simulink model "a01_SimTurret"  (R2024a)
settings: Solver=VariableStepAuto  StartTime=0.0  StopTime=10  FixedStep=0.000001  MaxStep=mSim.dTime*0.01  RelTol=mSim.dTime*0.01
PostLoadFcn:
  | a02_SimVariable
undefined symbols (not defined in the file): A02MTRPA, a1st, B01SCHED, b5th, C01ISENS, c7th, CRX1, DC, E03LIM, H01MDE, H01TRT, Init, mDefine, Mech, mSim, MtrPar, Sim, SIM, SimMde
libraries: spsSeriesRLCBranchLib x17, simulink x8, spsCurrentMeasurementLib x7, spsIGBTDiodeLib x7, spsDiodeLib x6, spsControlledVoltageSourceLib x6, spsVoltageMeasurementLib x4, SignalEditorBlockLib x3, spsDCVoltageSourceLib x1, spspowerguiLib x1
(part 2 of 3)

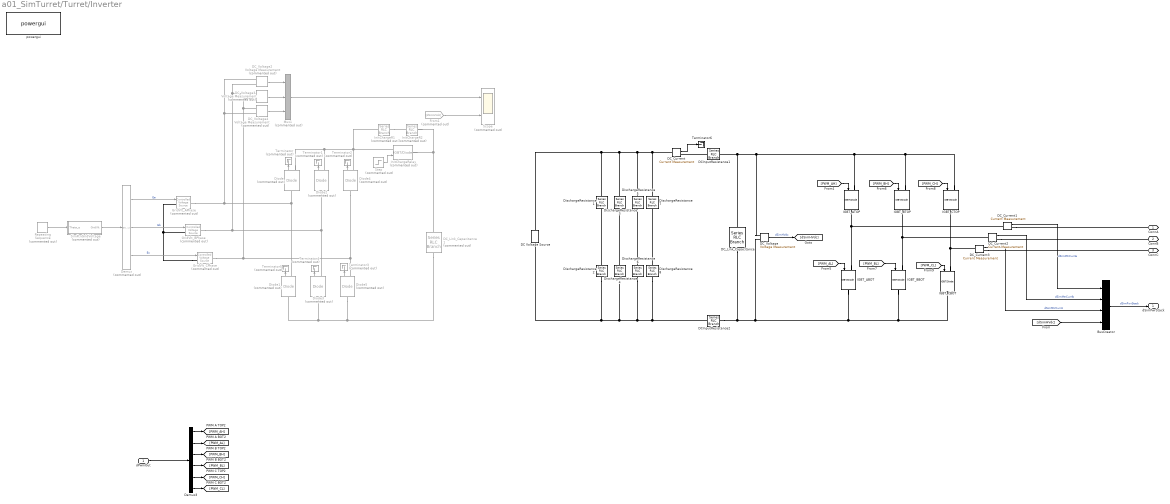
== system a01_SimTurret/Turret/Inverter ==
  dPwmOut : Inport
  BusCreator : BusCreator  Inputs=4
  DC Voltage Source : spsDCVoltageSourceLib/DC Voltage Source  Amplitude=Sim.dInitHVdc  Measurements=None
  DCInputResistance1 : spsSeriesRLCBranchLib/Series RLC Branch  LConnTagsString=__new0  RConnTagsString=__new0  BranchType=R  Resistance=1e-3  Inductance=1e-6  SetiL0=off  InitialCurrent=0  Capacitance=1e-6  Setx0=off  InitialVoltage=0  Measurements=None
  DCInputResistance2 : spsSeriesRLCBranchLib/Series RLC Branch  LConnTagsString=__new0  RConnTagsString=__new0  BranchType=R  Resistance=1e-3  Inductance=1e-6  SetiL0=off  InitialCurrent=0  Capacitance=1e-6  Setx0=off  InitialVoltage=0  Measurements=None
  DC_Current{,1..3} (4 alike) : spsCurrentMeasurementLib/Current Measurement  PhasorSimulation=off  OutputType=Complex  PSBequivalent=0
  DC_Link_Capacitance : spsSeriesRLCBranchLib/Series RLC Branch  LConnTagsString=__new0  RConnTagsString=__new0  BranchType=C  Resistance=DC.Rout  Inductance=1e-3  SetiL0=off  InitialCurrent=0  Capacitance=Sim.Dc.Capacitance  Setx0=on  InitialVoltage=Sim.dInitHVdc  Measurements=None
  DC_Link_Capacitance1 : spsSeriesRLCBranchLib/Series RLC Branch  Commented=on  LConnTagsString=__new0  RConnTagsString=__new0  BranchType=C  Resistance=DC.Rout  Inductance=1e-3  SetiL0=off  InitialCurrent=0  Capacitance=Sim.Dc.Capacitance  Setx0=on  InitialVoltage=Sim.dInitHVdc  Measurements=None
  DC_Voltage : spsVoltageMeasurementLib/Voltage Measurement  PhasorSimulation=off  OutputType=Complex  PSBequivalent=0
  DC_Voltage2 : spsVoltageMeasurementLib/Voltage Measurement  Commented=on  PhasorSimulation=off  OutputType=Complex  PSBequivalent=0
  DC_Voltage3 : spsVoltageMeasurementLib/Voltage Measurement  Commented=on  PhasorSimulation=off  OutputType=Complex  PSBequivalent=0
  DC_Voltage4 : spsVoltageMeasurementLib/Voltage Measurement  Commented=on  PhasorSimulation=off  OutputType=Complex  PSBequivalent=0
  Demux : Demux  Commented=on  Outputs=3
  Demux3 : Demux  Outputs=6
  Diode{,1..5} (6 alike) : spsDiodeLib/Diode  Commented=on  Ron=0.001  Lon=0  Vf=0.8  IC=0  UseSnubber=0  Rs=500  Cs=250e-9  Measurements=on
  DischargeResistance{1..8} (8 alike) : spsSeriesRLCBranchLib/Series RLC Branch  LConnTagsString=__new0  RConnTagsString=__new0  BranchType=R  Resistance=Sim.Dc.DischargeR  Inductance=1e-3  SetiL0=off  InitialCurrent=0  Capacitance=1e-6  Setx0=off  InitialVoltage=0  Measurements=None
  From1 : From  Commented=on  GotoTag=dSimHVdc
  GridVlt_APhase : spsControlledVoltageSourceLib/Controlled Voltage Source  Commented=on  Initialize=off  Source_Type=DC  Amplitude=0  Phase=0  Frequency=0  Measurements=None
  GridVlt_BPhase : spsControlledVoltageSourceLib/Controlled Voltage Source  Commented=on  Initialize=off  Source_Type=DC  Amplitude=0  Phase=0  Frequency=0  Measurements=None
  GridVlt_CPhase : spsControlledVoltageSourceLib/Controlled Voltage Source  Commented=on  Initialize=off  Source_Type=DC  Amplitude=0  Phase=0  Frequency=0  Measurements=None
  IGBT_ABOT : spsIGBTDiodeLib/IGBT//Diode  Ron=Sim.Igbt.Ron  Rs=Sim.Igbt.Roff  Cs=Sim.Igbt.Csnb  Measurements=off
  IGBT_ATOP : spsIGBTDiodeLib/IGBT//Diode  Ron=Sim.Igbt.Ron  Rs=Sim.Igbt.Roff  Cs=Sim.Igbt.Csnb  Measurements=off
  IGBT_BBOT : spsIGBTDiodeLib/IGBT//Diode  Ron=Sim.Igbt.Ron  Rs=Sim.Igbt.Roff  Cs=Sim.Igbt.Csnb  Measurements=off
  IGBT_BTOP : spsIGBTDiodeLib/IGBT//Diode  Ron=Sim.Igbt.Ron  Rs=Sim.Igbt.Roff  Cs=Sim.Igbt.Csnb  Measurements=off
  IGBT_CBOT : spsIGBTDiodeLib/IGBT//Diode  Ron=Sim.Igbt.Ron  Rs=Sim.Igbt.Roff  Cs=Sim.Igbt.Csnb  Measurements=off
  IGBT_CTOP : spsIGBTDiodeLib/IGBT//Diode  Ron=Sim.Igbt.Ron  Rs=Sim.Igbt.Roff  Cs=Sim.Igbt.Csnb  Measurements=off
  InitChargeR1 : spsSeriesRLCBranchLib/Series RLC Branch  Commented=on  LConnTagsString=__new0  RConnTagsString=__new0  BranchType=R  Resistance=Sim.Dc.InitChargeR  Inductance=1e-3  SetiL0=off  InitialCurrent=0  Capacitance=1e-6  Setx0=off  InitialVoltage=0  Measurements=None
  InitChargeR2 : spsSeriesRLCBranchLib/Series RLC Branch  Commented=on  LConnTagsString=__new0  RConnTagsString=__new0  BranchType=R  Resistance=Sim.Dc.InitChargeR  Inductance=1e-3  SetiL0=off  InitialCurrent=0  Capacitance=1e-6  Setx0=off  InitialVoltage=0  Measurements=None
  InitChargeRelay : spsIGBTDiodeLib/IGBT//Diode  Commented=on  Ron=Sim.Igbt.Ron  Rs=Sim.Igbt.Roff  Cs=Sim.Igbt.Csnb  Measurements=off
  Mux1 : Mux  Commented=on  Inputs=3
  Repeating Sequence : simulink/Sources/Repeating Sequence  Commented=on  rep_seq_t=[0 0.016666667]  rep_seq_y=[0 6.2832]
  Scope : Scope  Commented=on  NumInputPorts=2
  SimFtnGridVoltage : Subsystem  Commented=on  TreatAsAtomicUnit=on
  Step : Step  Commented=on  Time=0  SampleTime=0
  Terminator{,1..5} (6 alike) : Terminator  Commented=on
  Terminator6 : Terminator
  powergui : spspowerguiLib/powergui  Priority=1  SimulationMode=Continuous  SampleTime=50e-6  frequency=60  Iterations=50  frequencyindice=0  Pbase=100e6  ErrMax=1e-4  UnitsV=kV  UnitsW=MW  buscounter=0  FunctionMessages=off  echomessages=off  EnableUseOfTLC=off  CurrentSourceSwitches=off  DisableSnubberDevices=off  DisableRonSwitches=off  DisableVfSwitches=off  DisplayEquations=off  AutomaticDiscreteSolvers=off  SolverType=Tustin/Backward Euler (TBE)  Interpol=off  ExternalGateDelay=off  methode=off  Ts=100  x0status=blocks  SPID=on  SwTol=0  HookPort=off  NonlinearTolerance=1e-4  nMaxIteration=100  ContinueOnMaxIteration=off  RestoreLinks=warning  ResistiveCurrentMeasurement=off  Frange=[0:2:500]  Ylog=off  Xlog=on  ShowGrid=off  save=off  variable=ZData  structure=0  ZoomFFT=off  StartTime=0.0  cycles=1  DisplayStyle=1  fundamental=60  FreqAxis=off  MaxFrequency=1000  frequencyindicesteady=1  RmsSteady=1  display=off
  ConnA : PMIOPort  Side=Right
  ConnB : PMIOPort  Port=2  Side=Right
  ConnC : PMIOPort  Port=3  Side=Right
  dSimPwrStack : Outport
  wires:
  Demux3/2 -> [PWM_AL]
  [PWM_AL] -> IGBT_ABOT/1
  [PWM_BH] -> IGBT_BTOP/1
  [PWM_AH] -> IGBT_ATOP/1
  [PWM_CH] -> IGBT_CTOP/1
  [PWM_CL] -> IGBT_CBOT/1
  Demux3/1 -> [PWM_AH]
  dPwmOut/1 -> Demux3/1
  Demux3/3 -> [PWM_BH]
  Demux3/4 -> [PWM_BL]
  Demux3/5 -> [PWM_CH]
  Demux3/6 -> [PWM_CL]
  [PWM_BL] -> IGBT_BBOT/1
  DC_Voltage/1 -> [dSimHVdc]  "dSimHVdc"
  DC_Current1/1 -> BusCreator/1  "dSimMtrCurrIa"
  DC_Current2/1 -> BusCreator/2  "dSimMtrCurrIb"
  DC_Current3/1 -> BusCreator/3  "dSimMtrCurrIc"
  BusCreator/1 -> dSimPwrStack/1  "dSimPwrStack"
  Demux/2 -> GridVlt_BPhase/1  "Eb"
  Repeating Sequence/1 -> SimFtnGridVoltage/1(Theta_e)
  DC_Voltage2/1 -> Mux1/1
  DC_Voltage4/1 -> Mux1/3
  DC_Voltage3/1 -> Mux1/2
  Demux/3 -> GridVlt_CPhase/1  "Ec"
  Demux/1 -> GridVlt_APhase/1  "Ea"
  SimFtnGridVoltage/1(GridVlt) -> Demux/1
  Mux1/1 -> Scope/1
  Step/1 -> InitChargeRelay/1
  [dSimHVdc] -> BusCreator/4
  From1/1 -> Scope/2
  Diode/1 -> Terminator/1
  Diode2/1 -> Terminator1/1
  Diode4/1 -> Terminator2/1
  Diode3/1 -> Terminator4/1
  Diode1/1 -> Terminator5/1
  Diode5/1 -> Terminator3/1
  DC_Current/1 -> Terminator6/1
  connections:
  DC_Link_Capacitance/LConn1 -- DC_Voltage/LConn1 -- IGBT_CTOP/LConn1 -- IGBT_BTOP/LConn1 -- IGBT_ATOP/LConn1 -- DCInputResistance1/RConn1
  IGBT_ABOT/LConn1 -- IGBT_ATOP/RConn1 -- DC_Current1/LConn1
  IGBT_BBOT/LConn1 -- IGBT_BTOP/RConn1 -- DC_Current2/LConn1
  IGBT_CBOT/LConn1 -- IGBT_CTOP/RConn1 -- DC_Current3/LConn1
  DCInputResistance1/LConn1 -- DC_Current/RConn1
  DC_Current1/RConn1 -- ConnA/RConn1
  DC_Current2/RConn1 -- ConnB/RConn1
  DC_Current3/RConn1 -- ConnC/RConn1
  DC_Link_Capacitance/RConn1 -- DCInputResistance2/RConn1 -- DC_Voltage/LConn2 -- IGBT_BBOT/RConn1 -- IGBT_CBOT/RConn1 -- IGBT_ABOT/RConn1
  Diode1/RConn1 -- GridVlt_APhase/RConn1 -- DC_Voltage2/LConn1 -- DC_Voltage4/LConn2 -- Diode/LConn1
  Diode2/LConn1 -- Diode3/RConn1 -- GridVlt_BPhase/RConn1 -- DC_Voltage2/LConn2 -- DC_Voltage3/LConn1
  DC Voltage Source/LConn1 -- DCInputResistance2/LConn1 -- DischargeResistance8/LConn1 -- DischargeResistance6/LConn1 -- DischargeResistance4/LConn1 -- DischargeResistance2/LConn1
  DC_Voltage4/LConn1 -- GridVlt_CPhase/RConn1 -- Diode5/RConn1 -- Diode4/LConn1 -- DC_Voltage3/LConn2
  Diode/RConn1 -- Diode2/RConn1 -- InitChargeR1/LConn1 -- InitChargeRelay/LConn1 -- Diode4/RConn1
  GridVlt_CPhase/LConn1 -- GridVlt_APhase/LConn1 -- GridVlt_BPhase/LConn1
  InitChargeR2/RConn1 -- InitChargeRelay/RConn1 -- DC_Link_Capacitance1/LConn1
  InitChargeR1/RConn1 -- InitChargeR2/LConn1
  DischargeResistance2/RConn1 -- DischargeResistance1/LConn1
  DischargeResistance4/RConn1 -- DischargeResistance3/LConn1
  DischargeResistance6/RConn1 -- DischargeResistance5/LConn1
  DischargeResistance8/RConn1 -- DischargeResistance7/LConn1
  DC_Link_Capacitance1/RConn1 -- Diode1/LConn1 -- Diode3/LConn1 -- Diode5/LConn1
  DC_Current/LConn1 -- DischargeResistance7/RConn1 -- DischargeResistance3/RConn1 -- DischargeResistance1/RConn1 -- DC Voltage Source/RConn1 -- DischargeResistance5/RConn1

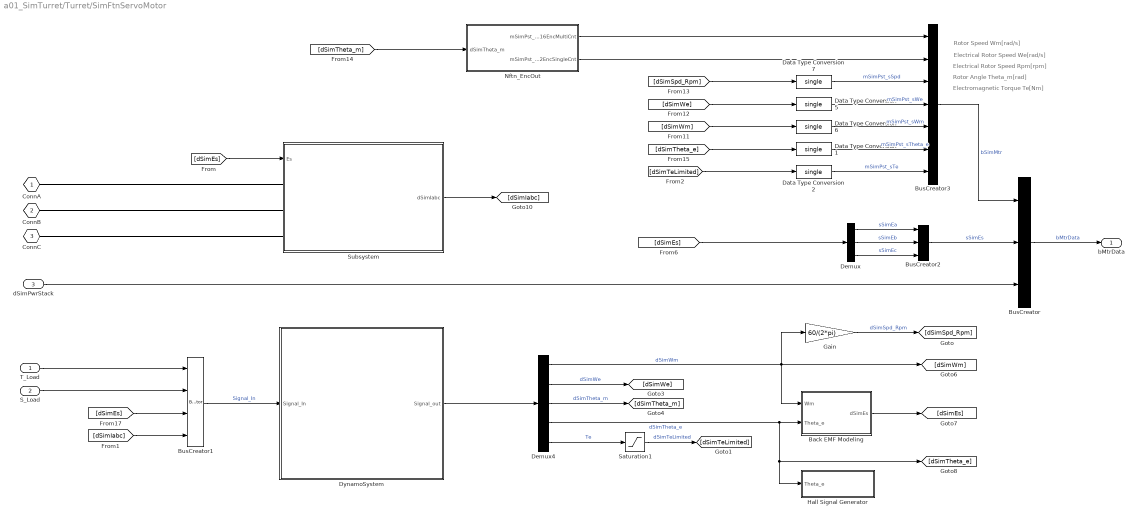
== system a01_SimTurret/Turret/SimFtnServoMotor ==
  note: Electromagnetic Torque Te[Nm]
  note: Rotor Angle Theta_m[rad]
  note: Electrical Rotor Speed Rpm[rpm]
  note: Electrical Rotor Speed We[rad/s]
  note: Rotor Speed Wm[rad/s]
  T_Load : Inport
  S_Load : Inport  Port=2
  dSimPwrStack : Inport  Port=3
  Back EMF Modeling : Subsystem
  BusCreator : BusCreator  Inputs=3
  BusCreator1 : BusCreator  Inputs=4
  BusCreator2 : BusCreator  Inputs=3
  BusCreator3 : BusCreator  Inputs=7
  Data Type Conversion{1..2,5..7} (5 alike) : DataTypeConversion  OutDataTypeStr=single  SaturateOnIntegerOverflow=off  RndMeth=Floor
  Demux : Demux  Outputs=3
  Demux4 : Demux  Outputs=5
  DynamoSystem : Subsystem  Variant=on
      mask Display: image('TorqueAndPowerCurves.png');
  Gain : Gain  Gain=60/(2*pi)
  Hall Signal Generator : Subsystem
  Nftn_EncOut : Subsystem
  Saturation1 : Saturate  UpperLimit=20  LowerLimit=-20
  Subsystem : Subsystem
      mask Display: image('Image09_Mtr_3.jpg');
  ConnA : PMIOPort  Side=Left
  ConnB : PMIOPort  Port=2  Side=Left
  ConnC : PMIOPort  Port=3  Side=Left
  bMtrData : Outport  VectorParamsAs1DForOutWhenUnconnected=off
  wires:
  [dSimWe] -> Data Type Conversion5/1
  [dSimWm] -> Data Type Conversion6/1
  [dSimEs] -> Demux/1
  Demux4/1 -> Back EMF Modeling/1(Wm), [dSimWm], Gain/1  "dSimWm"
  T_Load/1 -> BusCreator1/1
  DynamoSystem/1(Signal_out) -> Demux4/1
  [dSimTheta_e] -> Data Type Conversion1/1
  Demux4/3 -> [dSimTheta_m]  "dSimTheta_m"
  Demux4/2 -> [dSimWe]  "dSimWe"
  Data Type Conversion5/1 -> BusCreator3/4  "mSimPst_sWe"
  Subsystem/1(dSimIabc) -> [dSimIabc]
  Demux4/4 -> Hall Signal Generator/1(Theta_e), [dSimTheta_e], Back EMF Modeling/2(Theta_e)  "dSimTheta_e"
  BusCreator/1 -> bMtrData/1  "bMtrData"
  Back EMF Modeling/1(dSimEs) -> [dSimEs]
  [dSimEs] -> BusCreator1/3
  Demux4/5 -> Saturation1/1  "Te"
  S_Load/1 -> BusCreator1/2
  [dSimSpd_Rpm] -> Data Type Conversion7/1
  BusCreator3/1 -> BusCreator/1  "bSimMtr"
  [dSimEs] -> Subsystem/1(Es)
  BusCreator1/1 -> DynamoSystem/1(Signal_In)  "Signal_In"
  Gain/1 -> [dSimSpd_Rpm]  "dSimSpd_Rpm"
  Data Type Conversion6/1 -> BusCreator3/5  "mSimPst_sWm"
  Data Type Conversion7/1 -> BusCreator3/3  "mSimPst_sSpd"
  Saturation1/1 -> [dSimTeLimited]  "dSimTeLimited"
  [dSimIabc] -> BusCreator1/4
  dSimPwrStack/1 -> BusCreator/3
  Demux/2 -> BusCreator2/2  "sSimEb"
  Demux/1 -> BusCreator2/1  "sSimEa"
  Demux/3 -> BusCreator2/3  "sSimEc"
  BusCreator2/1 -> BusCreator/2  "sSimEs"
  Data Type Conversion1/1 -> BusCreator3/6  "mSimPst_sTheta_e"
  [dSimTeLimited] -> Data Type Conversion2/1
  Data Type Conversion2/1 -> BusCreator3/7  "mSimPst_sTe"
  [dSimTheta_m] -> Nftn_EncOut/1(dSimTheta_m)
  Nftn_EncOut/1(mSimPst_u16EncMultiCnt) -> BusCreator3/1
  Nftn_EncOut/2(mSimPst_u32EncSingleCnt) -> BusCreator3/2
  connections:
  ConnA/RConn1 -- Subsystem/LConn1
  Subsystem/LConn2 -- ConnB/RConn1
  Subsystem/LConn3 -- ConnC/RConn1

== system a01_SimTurret/Turret/SystemLoad ==
  bMtrData : Inport
  BusSelector : BusSelector  OutputSignals=bSimMtr.mSimPst_sSpd
  Constant1 : Constant  Value=1000  OutDataTypeStr=double
  Gain : Gain  Gain=0.002
  Saturation : Saturate  UpperLimit=E03LIM.sMaxTqSet  LowerLimit=E03LIM.sNegMaxTqSet
  T_Load : Outport
  S_Load : Outport  Port=2
  wires:
  Gain/1 -> Saturation/1  "T_LoadUlimited"
  Constant1/1 -> S_Load/1  "S_Load"
  bMtrData/1 -> BusSelector/1
  BusSelector/1 -> Gain/1  "<mSimPst_sSpd>"
  Saturation/1 -> T_Load/1  "T_Load"

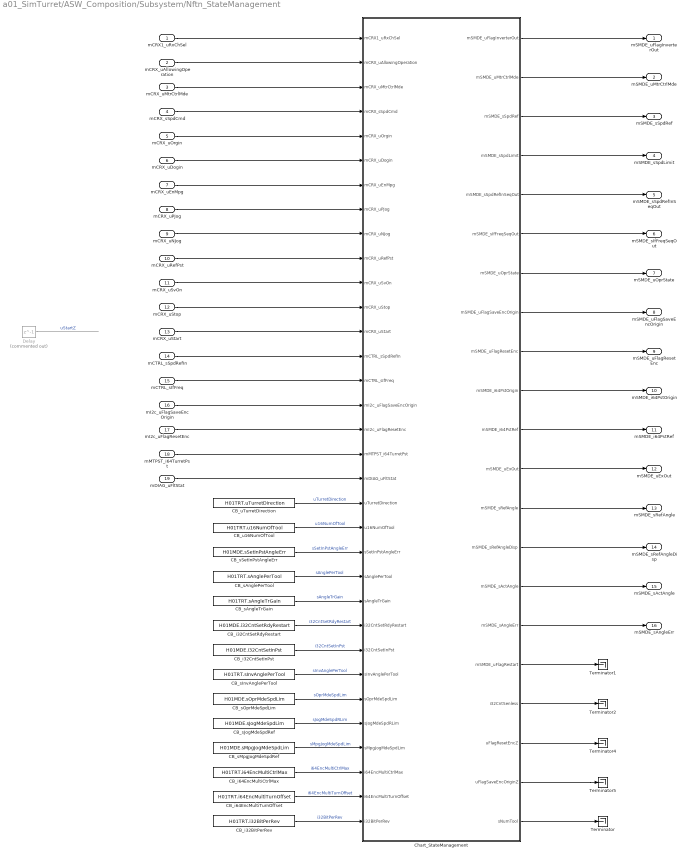
== system a01_SimTurret/ASW_Composition/Subsystem/Nftn_StateManagement ==
  mCRX1_uRxChSel : Inport
  mCRX_uAllowingOperation : Inport  Port=2
  mCRX_uMtrCtrlMde : Inport  Port=3
  mCRX_sSpdCmd : Inport  Port=4
  mCRX_uOrgin : Inport  Port=5
  mCRX_uDogin : Inport  Port=6
  mCRX_uEnMpg : Inport  Port=7
  mCRX_uPJog : Inport  Port=8
  mCRX_uNJog : Inport  Port=9
  mCRX_uRefPst : Inport  Port=10
  mCRX_uSvOn : Inport  Port=11
  mCRX_uStop : Inport  Port=12
  mCRX_uStart : Inport  Port=13
  mCTRL_sSpdRefIn : Inport  Port=14
  mCTRL_sIfFreq : Inport  Port=15
  mI2c_uFlagSaveEncOrigin : Inport  Port=16
  mI2c_uFlagResetEnc : Inport  Port=17
  mMTPST_i64TurretPst : Inport  Port=18
  mDIAG_uFltStat : Inport  Port=19
  CB_i32BitPerRev : Constant  Value=H01TRT.i32BitPerRev
  CB_i32CntSetInPst : Constant  Value=H01MDE.i32CntSetInPst
  CB_i32CntSetRdyRestart : Constant  Value=H01MDE.i32CntSetRdyRestart
  CB_i64EncMultiCtrlMax : Constant  Value=H01TRT.i64EncMultiCtrlMax
  CB_i64EncMultiTurnOffset : Constant  Value=H01TRT.i64EncMultiTurnOffset
  CB_sAnglePerTool : Constant  Value=H01TRT.sAnglePerTool
  CB_sAngleTrGain : Constant  Value=H01TRT.sAngleTrGain
  CB_sInvAnglePerTool : Constant  Value=H01TRT.sInvAnglePerTool
  CB_sJogMdeSpdRef : Constant  Value=H01MDE.sJogMdeSpdLim
  CB_sMpgJogMdeSpdRef : Constant  Value=H01MDE.sMpgJogMdeSpdLim
  CB_sOprMdeSpdLim : Constant  Value=H01MDE.sOprMdeSpdLim
  CB_sSetInPstAngleErr : Constant  Value=H01MDE.sSetInPstAngleErr
  CB_u16NumOfTool : Constant  Value=H01TRT.u16NumOfTool
  CB_uTurretDirection : Constant  Value=H01TRT.uTurretDirection
  Chart_StateManagement : Stateflow chart  TreatAsAtomicUnit=on
  Delay : Delay  Commented=on  DelayLength=1  StateName=uStart
  Terminator{,1..2,4..5} (5 alike) : Terminator
  mSMDE_uFlagInverterOut : Outport
  mSMDE_uMtrCtrlMde : Outport  Port=2
  mSMDE_sSpdRef : Outport  Port=3
  mSMDE_sSpdLimit : Outport  Port=4
  mSMDE_sSpdRefInSeqOut : Outport  Port=5
  mSMDE_sIfFreqSeqOut : Outport  Port=6
  mSMDE_uOprState : Outport  Port=7
  mSMDE_uFlagSaveEncOrigin : Outport  Port=8
  mSMDE_uFlagResetEnc : Outport  Port=9
  mSMDE_i64PstOrigin : Outport  Port=10
  mSMDE_i64PstRef : Outport  Port=11
  mSMDE_uExOut : Outport  Port=12
  mSMDE_sRefAngle : Outport  Port=13
  mSMDE_sRefAngleDisp : Outport  Port=14
  mSMDE_sActAngle : Outport  Port=15
  mSMDE_sAngleErr : Outport  Port=16
  wires:
  mCRX_uMtrCtrlMde/1 -> Chart_StateManagement/3(mCRX_uMtrCtrlMde)
  Chart_StateManagement/3(mSMDE_sSpdRef) -> mSMDE_sSpdRef/1
  Chart_StateManagement/5(mSMDE_sSpdRefInSeqOut) -> mSMDE_sSpdRefInSeqOut/1
  Chart_StateManagement/1(mSMDE_uFlagInverterOut) -> mSMDE_uFlagInverterOut/1
  mCRX_uAllowingOperation/1 -> Chart_StateManagement/2(mCRX_uAllowingOperation)
  Chart_StateManagement/6(mSMDE_sIfFreqSeqOut) -> mSMDE_sIfFreqSeqOut/1
  mCTRL_sSpdRefIn/1 -> Chart_StateManagement/14(mCTRL_sSpdRefIn)
  Chart_StateManagement/2(mSMDE_uMtrCtrlMde) -> mSMDE_uMtrCtrlMde/1
  mCTRL_sIfFreq/1 -> Chart_StateManagement/15(mCTRL_sIfFreq)
  mCRX_sSpdCmd/1 -> Chart_StateManagement/4(mCRX_sSpdCmd)
  mCRX1_uRxChSel/1 -> Chart_StateManagement/1(mCRX1_uRxChSel)
  Chart_StateManagement/7(mSMDE_uOprState) -> mSMDE_uOprState/1
  Chart_StateManagement/8(mSMDE_uFlagSaveEncOrigin) -> mSMDE_uFlagSaveEncOrigin/1
  Chart_StateManagement/10(mSMDE_i64PstOrigin) -> mSMDE_i64PstOrigin/1
  mCRX_uOrgin/1 -> Chart_StateManagement/5(mCRX_uOrgin)
  mCRX_uDogin/1 -> Chart_StateManagement/6(mCRX_uDogin)
  mI2c_uFlagSaveEncOrigin/1 -> Chart_StateManagement/16(mI2c_uFlagSaveEncOrigin)
  Chart_StateManagement/9(mSMDE_uFlagResetEnc) -> mSMDE_uFlagResetEnc/1
  mI2c_uFlagResetEnc/1 -> Chart_StateManagement/17(mI2c_uFlagResetEnc)
  Chart_StateManagement/11(mSMDE_i64PstRef) -> mSMDE_i64PstRef/1
  mCRX_uEnMpg/1 -> Chart_StateManagement/7(mCRX_uEnMpg)
  mCRX_uPJog/1 -> Chart_StateManagement/8(mCRX_uPJog)
  mCRX_uNJog/1 -> Chart_StateManagement/9(mCRX_uNJog)
  mMTPST_i64TurretPst/1 -> Chart_StateManagement/18(mMTPST_i64TurretPst)
  mCRX_uStart/1 -> Chart_StateManagement/13(mCRX_uStart)
  Delay/1 -> ?  "uStartZ"
  mCRX_uRefPst/1 -> Chart_StateManagement/10(mCRX_uRefPst)
  CB_sAnglePerTool/1 -> Chart_StateManagement/23(sAnglePerTool)  "sAnglePerTool"
  Chart_StateManagement/13(mSMDE_sRefAngle) -> mSMDE_sRefAngle/1
  CB_u16NumOfTool/1 -> Chart_StateManagement/21(u16NumOfTool)  "u16NumOfTool"
  Chart_StateManagement/12(mSMDE_uExOut) -> mSMDE_uExOut/1
  mDIAG_uFltStat/1 -> Chart_StateManagement/19(mDIAG_uFltStat)
  CB_i32CntSetRdyRestart/1 -> Chart_StateManagement/25(i32CntSetRdyRestart)  "i32CntSetRdyRestart"
  Chart_StateManagement/17(mSMDE_uFlagRestart) -> Terminator1/1
  Chart_StateManagement/18(i32CntSenless) -> Terminator2/1
  CB_sAngleTrGain/1 -> Chart_StateManagement/24(sAngleTrGain)  "sAngleTrGain"
  Chart_StateManagement/15(mSMDE_sActAngle) -> mSMDE_sActAngle/1
  Chart_StateManagement/19(uFlagResetEncZ) -> Terminator4/1
  Chart_StateManagement/20(uFlagSaveEncOriginZ) -> Terminator5/1
  mCRX_uSvOn/1 -> Chart_StateManagement/11(mCRX_uSvOn)
  CB_uTurretDirection/1 -> Chart_StateManagement/20(uTurretDirection)  "uTurretDirection"
  Chart_StateManagement/16(mSMDE_sAngleErr) -> mSMDE_sAngleErr/1
  CB_sSetInPstAngleErr/1 -> Chart_StateManagement/22(sSetInPstAngleErr)  "sSetInPstAngleErr"
  CB_i32CntSetInPst/1 -> Chart_StateManagement/26(i32CntSetInPst)  "i32CntSetInPst"
  mCRX_uStop/1 -> Chart_StateManagement/12(mCRX_uStop)
  CB_sInvAnglePerTool/1 -> Chart_StateManagement/27(sInvAnglePerTool)  "sInvAnglePerTool"
  CB_sJogMdeSpdRef/1 -> Chart_StateManagement/29(sJogMdeSpdRLim)  "sJogMdeSpdRLim"
  CB_sMpgJogMdeSpdRef/1 -> Chart_StateManagement/30(sMpgJogMdeSpdLim)  "sMpgJogMdeSpdLim"
  CB_i64EncMultiCtrlMax/1 -> Chart_StateManagement/31(i64EncMultiCtrlMax)  "i64EncMultiCtrlMax"
  CB_i64EncMultiTurnOffset/1 -> Chart_StateManagement/32(i64EncMultiTurnOffset)  "i64EncMultiTurnOffset"
  CB_i32BitPerRev/1 -> Chart_StateManagement/33(i32BitPerRev)  "i32BitPerRev"
  Chart_StateManagement/4(mSMDE_sSpdLimit) -> mSMDE_sSpdLimit/1
  Chart_StateManagement/21(sNumTool) -> Terminator/1
  CB_sOprMdeSpdLim/1 -> Chart_StateManagement/28(sOprMdeSpdLim)  "sOprMdeSpdLim"
  Chart_StateManagement/14(mSMDE_sRefAngleDisp) -> mSMDE_sRefAngleDisp/1

== system a01_SimTurret/Subsystem/Ftn_MtrCtrlPwmSet/PWM_DEFAULT ==
  bTBC : Inport
  ActionPort : ActionPort  ActionPortLabel=else
  Bus Selector : BusSelector  OutputSignals=uPrd
  Constant : Constant  Value=0  OutDataTypeStr=uint16
  Mux : Mux  Inputs=6
  PWM_OUT : Outport  VectorParamsAs1DForOutWhenUnconnected=off
  wires:
  Constant/1 -> Mux/1, Mux/3, Mux/5  "u16Zero"
  Mux/1 -> PWM_OUT/1  "PWM_OUT"
  bTBC/1 -> Bus Selector/1
  Bus Selector/1 -> Mux/2, Mux/4, Mux/6  "<uPrd>"

== system a01_SimTurret/Subsystem/Ftn_MtrCtrlPwmSet/PWM_FOUT ==
  bE04GPWM : Inport
  bC01MADC : Inport  Port=2
  bTBC : Inport  Port=3
  ActionPort : ActionPort  ActionPortLabel=if(u1 == 1)
  Add : Sum
  Bus Selector1 : BusSelector  OutputSignals=uPrd,uPrdHalf
  BusSelector : BusSelector  OutputSignals=mGPwm_sVanRef,mGPwm_sVbnRef,mGPwm_sVcnRef
  BusSelector1 : BusSelector  OutputSignals=mMsens_sInvHVdcLow
  Constant : Constant  OutDataTypeStr=uint16
  Data Type Conversion : DataTypeConversion  OutDataTypeStr=single  SaturateOnIntegerOverflow=off  RndMeth=Floor
  Data Type Conversion1 : DataTypeConversion  OutDataTypeStr=single  SaturateOnIntegerOverflow=off  RndMeth=Floor
  Data Type Conversion2 : DataTypeConversion  OutDataTypeStr=uint16  SaturateOnIntegerOverflow=off  RndMeth=Floor
  Data Type Conversion3 : DataTypeConversion  OutDataTypeStr=uint16  SaturateOnIntegerOverflow=off  RndMeth=Floor
  Data Type Conversion4 : DataTypeConversion  OutDataTypeStr=uint16  SaturateOnIntegerOverflow=off  RndMeth=Floor
  Divide : Product  Inputs=**
  Mux : Mux  Inputs=6
  Mux1 : Mux  Inputs=3
  Product : Product
  Product1 : Product
  Product2 : Product
  Sum : Sum  Inputs=|++
  Sum1 : Sum  Inputs=|++
  Sum2 : Sum  Inputs=|++
  uPwmCompVal : Outport
  PWM_OUT : Outport  Port=2  VectorParamsAs1DForOutWhenUnconnected=off
  wires:
  bC01MADC/1 -> BusSelector1/1
  Divide/1 -> Product1/2, Product/2, Product2/2  "temp_f"
  BusSelector/1 -> Product/1  "<mGPwm_sVanRef>"
  BusSelector/3 -> Product2/1  "<mGPwm_sVcnRef>"
  BusSelector/2 -> Product1/1  "<mGPwm_sVbnRef>"
  Product/1 -> Sum/1
  Mux/1 -> PWM_OUT/1  "PWM_OUT"
  Product2/1 -> Sum2/1
  Product1/1 -> Sum1/1
  Bus Selector1/1 -> Data Type Conversion/1  "<uPrd>"
  Data Type Conversion1/1 -> Sum/2, Sum1/2, Sum2/2
  Data Type Conversion/1 -> Divide/2
  bE04GPWM/1 -> BusSelector/1
  bTBC/1 -> Bus Selector1/1
  Mux1/1 -> uPwmCompVal/1  "uPwmCompVal"
  Bus Selector1/2 -> Add/1  "<uPrdHalf>"
  Data Type Conversion2/1 -> Mux1/1, Mux/2, Mux/1
  Data Type Conversion4/1 -> Mux1/3, Mux/6, Mux/5
  Add/1 -> Data Type Conversion1/1
  Constant/1 -> Add/2
  Sum/1 -> Data Type Conversion2/1  "PwmCompU"
  Sum2/1 -> Data Type Conversion4/1  "PwmCompW"
  Sum1/1 -> Data Type Conversion3/1  "PwmCompV"
  Data Type Conversion3/1 -> Mux/4, Mux1/2, Mux/3
  BusSelector1/1 -> Divide/1  "<mMsens_sInvHVdcLow>"

== system a01_SimTurret/Turret/Inverter/SimFtnGridVoltage ==
  Theta_e : Inport
  -2PI/3 Phase Shift : Fcn  Expr=u(1) - 2*pi/3
  2PI/3 Phase Shift : Fcn  Expr=u(1) + 2*pi/3
  A Phase Back-EMF : Fcn  Expr=-sin(u(1))
  B Phase Back-EMF : Fcn  Expr=-sin(u(1))
  C Phase Back-EMF : Fcn  Expr=-sin(u(1))
  Constant : Constant  Value=Sim.dAcInputVlt*1.4212135/1.7372
  Mux : Mux  Inputs=3
  Product : Product
  GridVlt : Outport  VectorParamsAs1DForOutWhenUnconnected=off
  wires:
  Product/1 -> GridVlt/1
  Constant/1 -> Product/2
  B Phase Back-EMF/1 -> Mux/2  "Eb"
  A Phase Back-EMF/1 -> Mux/1  "Ea"
  C Phase Back-EMF/1 -> Mux/3  "Ec"
  -2PI/3 Phase Shift/1 -> B Phase Back-EMF/1  "Theta_e - 2PI/3"
  Mux/1 -> Product/1
  2PI/3 Phase Shift/1 -> C Phase Back-EMF/1  "Ttheta_e + 2PI/3"
  Theta_e/1 -> -2PI/3 Phase Shift/1, 2PI/3 Phase Shift/1, A Phase Back-EMF/1  "Theta_e"

== system a01_SimTurret/Turret/SimFtnServoMotor/Back EMF Modeling ==
  Wm : Inport
  Theta_e : Inport  Port=2
  AtcBackBemf : Subsystem  Commented=on  TreatAsAtomicUnit=on
  BackBemfShapeSelection : Constant  Value=Sim.Bemf.Set
  BemfConstant : Gain  Gain=MtrPar.Ke
  IdealTrapezoidalBackBemf : Subsystem  TreatAsAtomicUnit=on
  Merge : Merge  Inputs=4
  Product : Product
  SinewaveBackBemf : Subsystem  TreatAsAtomicUnit=on
  Step7thTrapezoidalBackBemf : Subsystem  TreatAsAtomicUnit=on
  Switch Case : SwitchCase  CaseConditions={0, 1, 2, 3}
  Terminator : Terminator
  dSimEs : Outport  VectorParamsAs1DForOutWhenUnconnected=off
  wires:
  Theta_e/1 -> AtcBackBemf/1(Theta_e), Step7thTrapezoidalBackBemf/1(Theta_e), IdealTrapezoidalBackBemf/1(Theta_e), SinewaveBackBemf/1(Theta_e)
  Switch Case/1 -> SinewaveBackBemf/Action  "Sinwave Back-EMF (Kind = 0)"
  Switch Case/2 -> IdealTrapezoidalBackBemf/Action  "Ideal Trapezoidal Back-EMF (Kind = 1)"
  IdealTrapezoidalBackBemf/1(Es) -> Merge/2  "Ideal Trapezoidal"
  Switch Case/3 -> Step7thTrapezoidalBackBemf/Action  "Step 7th Trapezoidal Back-EMF (Kind = 2)"
  Step7thTrapezoidalBackBemf/1(Es) -> Merge/3  "Step 7th Trapezoidal"
  Merge/1 -> Product/1  "MerOut"
  Product/1 -> dSimEs/1  "dSimEs"
  Switch Case/5 -> Terminator/1
  BackBemfShapeSelection/1 -> Switch Case/1
  SinewaveBackBemf/1(Es) -> Merge/1  "Sinewave"
  AtcBackBemf/1(Es) -> Merge/4  "eCOMP Back EMF"
  Switch Case/4 -> AtcBackBemf/Action  "System Back-EMF (Kind = 3)"
  Wm/1 -> BemfConstant/1
  BemfConstant/1 -> Product/2

== system a01_SimTurret/Turret/SimFtnServoMotor/DynamoSystem ==
  note: 1) Add Subsystem or Model blocks as valid variant choices.
      | 2) You cannot connect blocks at this level. At simulation, connectivity is automatically
      | determined, based on the active variant and port name matching.
  Signal_In : Inport
  SpeedMode : Subsystem  VariantControl=VrntDynamoMdeS0T1 == 0
  TorqueMode : Subsystem  VariantControl=VrntDynamoMdeS0T1 == 1
  Signal_out : Outport

== system a01_SimTurret/Turret/SimFtnServoMotor/Hall Signal Generator ==
  Theta_e : Inport
  -2PI/3 Phase Shift : Fcn  Expr=u(1) - 2*pi/3
  2PI/3 Phase Shift : Fcn  Expr=u(1) + 2*pi/3
  A Phase Hall Signal : Fcn  Expr=(0 <= u(1))*(u(1) < pi/6) + (7*pi/6 <= u(1))*(u(1) < 2*pi)
  B Phase Hall Signal : Fcn  Expr=(0 <= u(1))*(u(1) < pi/6) + (7*pi/6 <= u(1))*(u(1) < 2*pi)
  C Phase Hall Signal : Fcn  Expr=(0 <= u(1))*(u(1) < pi/6) + (7*pi/6 <= u(1))*(u(1) < 2*pi)
  Mux : Mux  Inputs=3
  Terminator : Terminator
  mode #1 : Fcn  Expr=u(1) - floor(u(1)/2/pi)*2*pi
  mode #2 : Fcn  Expr=u(1) - floor(u(1)/2/pi)*2*pi
  wires:
  mode #2/1 -> C Phase Hall Signal/1  "Theta_e + 2PI/3"
  Theta_e/1 -> 2PI/3 Phase Shift/1, A Phase Hall Signal/1, -2PI/3 Phase Shift/1
  2PI/3 Phase Shift/1 -> mode #2/1
  -2PI/3 Phase Shift/1 -> mode #1/1
  mode #1/1 -> B Phase Hall Signal/1  "Theta_e - 2PI/3"
  C Phase Hall Signal/1 -> Mux/3  "Hall C"
  B Phase Hall Signal/1 -> Mux/2  "Hall B"
  A Phase Hall Signal/1 -> Mux/1  "Hall A"
  Mux/1 -> Terminator/1  "dSimHall"

== system a01_SimTurret/Turret/SimFtnServoMotor/Nftn_EncOut ==
  dSimTheta_m : Inport
  Add : Sum
  Chart_EncOut : Stateflow chart  TreatAsAtomicUnit=on
  Constant : Constant  Value=mDefine.dEncoderPPR
  Constant1 : Constant  Value=0  OutDataTypeStr=single
  Constant2 : Constant  Value=2*pi
  DataTypeConversion3 : DataTypeConversion  OutDataTypeStr=int32  SaturateOnIntegerOverflow=off  RndMeth=Floor
  DataTypeConversion4 : DataTypeConversion  OutDataTypeStr=uint32  SaturateOnIntegerOverflow=off  RndMeth=Floor
  DataTypeConversion5 : DataTypeConversion  OutDataTypeStr=uint16  SaturateOnIntegerOverflow=off  RndMeth=Floor
  Divide : Product  Inputs=*/
  Product : Product
  Terminator : Terminator
  mod : Subsystem
  mSimPst_u16EncMultiCnt : Outport
  mSimPst_u32EncSingleCnt : Outport  Port=2
  wires:
  Constant1/1 -> Add/2
  DataTypeConversion4/1 -> mSimPst_u32EncSingleCnt/1  "mSimPst_u32EncSingleCnt"
  DataTypeConversion3/1 -> DataTypeConversion4/1, Chart_EncOut/1(i32EncSingleCnt)  "i32EncSingleCnt"
  Constant/1 -> Divide/1
  Divide/1 -> Product/2
  Constant2/1 -> Divide/2
  Add/1 -> mod/1(sThetaIntegIn)
  Chart_EncOut/1(i32EncMultiCnt) -> DataTypeConversion5/1
  mod/1(sThetaIntegOut) -> Product/1
  dSimTheta_m/1 -> Add/1
  Product/1 -> DataTypeConversion3/1
  DataTypeConversion5/1 -> mSimPst_u16EncMultiCnt/1  "mSimPst_u16EncMultiCnt"
  Chart_EncOut/2(i32EncSingleCntZ) -> Terminator/1

== system a01_SimTurret/Turret/SimFtnServoMotor/Subsystem ==
  Es : Inport
  APhase_Rs_Ls : spsSeriesRLCBranchLib/Series RLC Branch  LConnTagsString=__new0  RConnTagsString=__new0  BranchType=RL  Resistance=A02MTRPA.sRs  Inductance=A02MTRPA.sLs  SetiL0=off  InitialCurrent=Init(3)  Capacitance=1e-6  Setx0=off  InitialVoltage=0  Measurements=None
  A_Phase_BEMF : spsControlledVoltageSourceLib/Controlled Voltage Source  Initialize=off  Source_Type=DC  Amplitude=0  Phase=0  Frequency=0  Measurements=None
  BPhase_Rs_Ls : spsSeriesRLCBranchLib/Series RLC Branch  LConnTagsString=__new0  RConnTagsString=__new0  BranchType=RL  Resistance=A02MTRPA.sRs  Inductance=A02MTRPA.sLs  SetiL0=off  InitialCurrent=Init(3)  Capacitance=1e-6  Setx0=off  InitialVoltage=0  Measurements=None
  B_Phase_BEMF : spsControlledVoltageSourceLib/Controlled Voltage Source  Initialize=off  Source_Type=DC  Amplitude=0  Phase=0  Frequency=0  Measurements=None
  CPhase_Rs_Ls : spsSeriesRLCBranchLib/Series RLC Branch  LConnTagsString=__new0  RConnTagsString=__new0  BranchType=RL  Resistance=A02MTRPA.sRs  Inductance=A02MTRPA.sLs  SetiL0=off  InitialCurrent=Init(3)  Capacitance=1e-6  Setx0=off  InitialVoltage=0  Measurements=None
  C_Phase_BEMF : spsControlledVoltageSourceLib/Controlled Voltage Source  Initialize=off  Source_Type=DC  Amplitude=0  Phase=0  Frequency=0  Measurements=None
  Demux : Demux  Outputs=3
  Isens_Ia : spsCurrentMeasurementLib/Current Measurement  PhasorSimulation=off  OutputType=Complex  PSBequivalent=0
  Isens_Ib : spsCurrentMeasurementLib/Current Measurement  PhasorSimulation=off  OutputType=Complex  PSBequivalent=0
  Isens_Ic : spsCurrentMeasurementLib/Current Measurement  PhasorSimulation=off  OutputType=Complex  PSBequivalent=0
  Mux : Mux  Inputs=3
  ConnA : PMIOPort  Side=Left
  ConnB : PMIOPort  Port=2  Side=Left
  ConnC : PMIOPort  Port=3  Side=Left
  dSimIabc : Outport
  wires:
  Isens_Ib/1 -> Mux/2  "dSimIb"
  Isens_Ic/1 -> Mux/3  "dSimIc"
  Demux/3 -> C_Phase_BEMF/1  "Ec"
  Demux/1 -> A_Phase_BEMF/1  "Ea"
  Demux/2 -> B_Phase_BEMF/1  "Eb"
  Isens_Ia/1 -> Mux/1  "dSimIa"
  Es/1 -> Demux/1
  Mux/1 -> dSimIabc/1  "dSimIabc"
  connections:
  CPhase_Rs_Ls/RConn1 -- Isens_Ic/LConn1
  Isens_Ia/RConn1 -- A_Phase_BEMF/RConn1
  ConnA/RConn1 -- APhase_Rs_Ls/LConn1
  Isens_Ic/RConn1 -- C_Phase_BEMF/RConn1
  A_Phase_BEMF/LConn1 -- B_Phase_BEMF/LConn1 -- C_Phase_BEMF/LConn1
  APhase_Rs_Ls/RConn1 -- Isens_Ia/LConn1
  BPhase_Rs_Ls/LConn1 -- ConnB/RConn1
  Isens_Ib/RConn1 -- B_Phase_BEMF/RConn1
  BPhase_Rs_Ls/RConn1 -- Isens_Ib/LConn1
  CPhase_Rs_Ls/LConn1 -- ConnC/RConn1

== system a01_SimTurret/Turret/SimFtnServoMotor/Back EMF Modeling/AtcBackBemf ==
  Theta_e : Inport
  ActionPort : ActionPort
  APhaseBackBemf : Fcn  Expr=-1*(a1st*sin(u(1)) + b5th*sin(5*(u(1))) + c7th*sin(7*(u(1))))
  BPhaseBackBemf : Fcn  Expr=-1*(a1st*sin(u(1)) + b5th*sin(5*(u(1))) + c7th*sin(7*(u(1))))
  CPhaseBackBemf : Fcn  Expr=-1*(a1st*sin(u(1)) + b5th*sin(5*(u(1))) + c7th*sin(7*(u(1))))
  Mux : Mux  Inputs=3
  VPhaseShift : Fcn  Expr=u(1) - 2*pi/3
  WPhaseShift : Fcn  Expr=u(1) + 2*pi/3
  Es : Outport  VectorParamsAs1DForOutWhenUnconnected=off
  wires:
  WPhaseShift/1 -> CPhaseBackBemf/1  "Ttheta_e + 2PI/3"
  VPhaseShift/1 -> BPhaseBackBemf/1  "Theta_e - 2PI/3"
  Theta_e/1 -> WPhaseShift/1, VPhaseShift/1, APhaseBackBemf/1  "Theta_e"
  APhaseBackBemf/1 -> Mux/1  "Ea"
  BPhaseBackBemf/1 -> Mux/2  "Eb"
  CPhaseBackBemf/1 -> Mux/3  "Ec"
  Mux/1 -> Es/1

== system a01_SimTurret/Turret/SimFtnServoMotor/Back EMF Modeling/IdealTrapezoidalBackBemf ==
  Theta_e : Inport
  Action Port : ActionPort  ActionPortLabel=case [ 1 ]:
  -2PI/3 Phase Shift : Fcn  Expr=u(1) - 2*pi/3
  2PI/3 Phase Shift : Fcn  Expr=u(1) + 2*pi/3
  A Phase Back-EMF : Fcn  Expr=(0 <= u(1))*(u(1) < pi/6)*(-6/pi * u(1)) + (pi/6 <= u(1))*(u(1) < 5*pi/6)*(-1) + (5*pi/6 <= u(1))*(u(1) < 7*pi/6)*(6/pi * u(1) - 6) + (7*pi/6 <= u(1))*(u(1) < 11*pi/6)*(1) + (11*pi/6 <= u(1))*(u(1) < 2*pi)*(-6/pi * u(1) + 12)
  B Phase Back-EMF : Fcn  Expr=(0 <= u(1))*(u(1) < pi/6)*(-6/pi * u(1)) + (pi/6 <= u(1))*(u(1) < 5*pi/6)*(-1) + (5*pi/6 <= u(1))*(u(1) < 7*pi/6)*(6/pi * u(1) - 6) + (7*pi/6 <= u(1))*(u(1) < 11*pi/6)*(1) + (11*pi/6 <= u(1))*(u(1) < 2*pi)*(-6/pi * u(1) + 12)
  C Phase Back-EMF : Fcn  Expr=(0 <= u(1))*(u(1) < pi/6)*(-6/pi * u(1)) + (pi/6 <= u(1))*(u(1) < 5*pi/6)*(-1) + (5*pi/6 <= u(1))*(u(1) < 7*pi/6)*(6/pi * u(1) - 6) + (7*pi/6 <= u(1))*(u(1) < 11*pi/6)*(1) + (11*pi/6 <= u(1))*(u(1) < 2*pi)*(-6/pi * u(1) + 12)
  Mux : Mux  Inputs=3
  mode #1 : Fcn  Expr=u(1) - floor(u(1)/2/pi)*2*pi
  mode #2 : Fcn  Expr=u(1) - floor(u(1)/2/pi)*2*pi
  Es : Outport  VectorParamsAs1DForOutWhenUnconnected=off
  wires:
  Mux/1 -> Es/1
  C Phase Back-EMF/1 -> Mux/3  "Ec"
  B Phase Back-EMF/1 -> Mux/2  "Eb"
  A Phase Back-EMF/1 -> Mux/1  "Ea"
  Theta_e/1 -> 2PI/3 Phase Shift/1, -2PI/3 Phase Shift/1, A Phase Back-EMF/1  "Theta_e"
  -2PI/3 Phase Shift/1 -> mode #1/1
  2PI/3 Phase Shift/1 -> mode #2/1
  mode #1/1 -> B Phase Back-EMF/1  "Theta_e - 2*pi/3"
  mode #2/1 -> C Phase Back-EMF/1  "Theta_e + 2*pi/3"

== system a01_SimTurret/Turret/SimFtnServoMotor/Back EMF Modeling/SinewaveBackBemf ==
  Theta_e : Inport
  Action Port : ActionPort  ActionPortLabel=case [ 0 ]:
  -2PI/3 Phase Shift : Fcn  Expr=u(1) - 2*pi/3
  2PI/3 Phase Shift : Fcn  Expr=u(1) + 2*pi/3
  A Phase Back-EMF : Fcn  Expr=-sin(u(1))
  B Phase Back-EMF : Fcn  Expr=-sin(u(1))
  C Phase Back-EMF : Fcn  Expr=-sin(u(1))
  Mux : Mux  Inputs=3
  Es : Outport  VectorParamsAs1DForOutWhenUnconnected=off
  wires:
  2PI/3 Phase Shift/1 -> C Phase Back-EMF/1  "Ttheta_e + 2PI/3"
  -2PI/3 Phase Shift/1 -> B Phase Back-EMF/1  "Theta_e - 2PI/3"
  Theta_e/1 -> -2PI/3 Phase Shift/1, 2PI/3 Phase Shift/1, A Phase Back-EMF/1  "Theta_e"
  A Phase Back-EMF/1 -> Mux/1  "Ea"
  B Phase Back-EMF/1 -> Mux/2  "Eb"
  C Phase Back-EMF/1 -> Mux/3  "Ec"
  Mux/1 -> Es/1

== system a01_SimTurret/Turret/SimFtnServoMotor/Back EMF Modeling/Step7thTrapezoidalBackBemf ==
  Theta_e : Inport
  Action Port : ActionPort  ActionPortLabel=case [ 2 ]:
  -2PI/3 Phase Shift : Fcn  Expr=u(1) - 2*pi/3
  2PI/3 Phase Shift : Fcn  Expr=u(1) + 2*pi/3
  A Phase Back-EMF : Fcn  Expr=-1.2626*sin(u(1)) - 0.3931*sin(3*u(1)) - 0.2045*sin(5*u(1)) - 0.1158*sin(7*u(1))
  B Phase Back-EMF : Fcn  Expr=-1.2626*sin(u(1)) - 0.3931*sin(3*u(1)) - 0.2045*sin(5*u(1)) - 0.1158*sin(7*u(1))
  C Phase Back-EMF : Fcn  Expr=-1.2626*sin(u(1)) - 0.3931*sin(3*u(1)) - 0.2045*sin(5*u(1)) - 0.1158*sin(7*u(1))
  Mux : Mux  Inputs=3
  Es : Outport  VectorParamsAs1DForOutWhenUnconnected=off
  wires:
  2PI/3 Phase Shift/1 -> C Phase Back-EMF/1  "Ttheta_e + 2PI/3"
  -2PI/3 Phase Shift/1 -> B Phase Back-EMF/1  "Theta_e - 2PI/3"
  Theta_e/1 -> 2PI/3 Phase Shift/1, -2PI/3 Phase Shift/1, A Phase Back-EMF/1  "Theta_e"
  A Phase Back-EMF/1 -> Mux/1  "Ea"
  B Phase Back-EMF/1 -> Mux/2  "Eb"
  C Phase Back-EMF/1 -> Mux/3  "Ec"
  Mux/1 -> Es/1

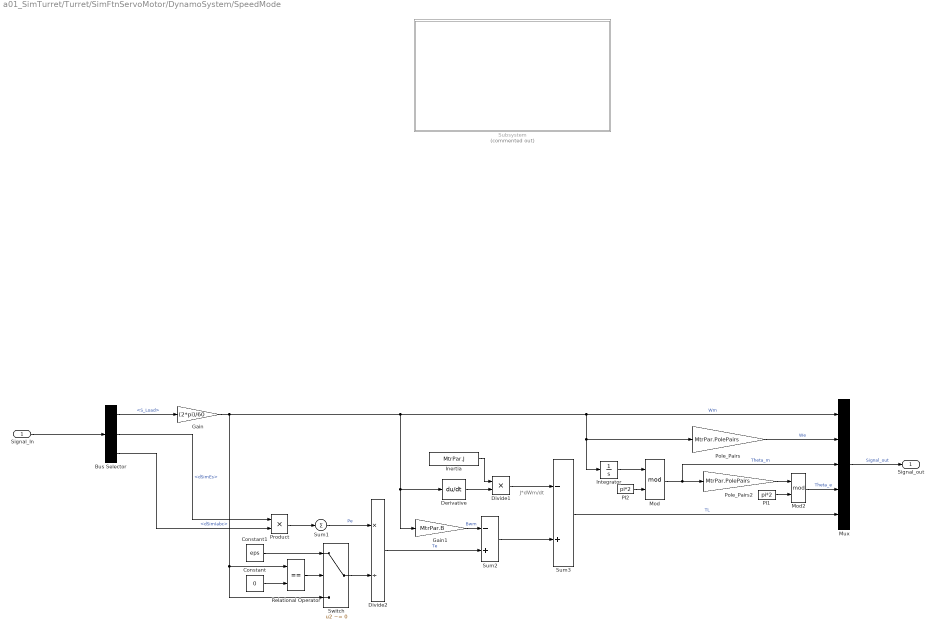
== system a01_SimTurret/Turret/SimFtnServoMotor/DynamoSystem/SpeedMode ==
  note: J*dWm/dt
  Signal_In : Inport
  Bus Selector : BusSelector  OutputSignals=S_Load,dSimEs,dSimIabc
  Constant : Constant  Value=0  OutDataTypeStr=double
  Constant1 : Constant  Value=eps  OutDataTypeStr=double
  Derivative : Derivative
  Divide1 : Product  Inputs=**
  Divide2 : Product  Inputs=*/
  Gain : Gain  Gain=(2*pi)/60
  Gain1 : Gain  Gain=MtrPar.B
  Inertia : Constant  Value=MtrPar.J
  Integrator : Integrator
  Mod : Math  Operator=mod  SignedPower=on
  Mod2 : Math  Operator=mod  SignedPower=on
  Mux : Mux  Inputs=5
  PI1 : Constant  Value=pi*2
  PI2 : Constant  Value=pi*2
  Pole_Pairs : Gain  Gain=MtrPar.PolePairs
  Pole_Pairs2 : Gain  Gain=MtrPar.PolePairs
  Product : Product
  Relational Operator : RelationalOperator  Operator===  OutDataTypeStr=boolean  RndMeth=Simplest  InputSameDT=off
  Subsystem : Subsystem  Commented=on
  Sum1 : Sum  Inputs=+
  Sum2 : Sum  Inputs=-+
  Sum3 : Sum  Inputs=-+
  Switch : Switch  Criteria=u2 ~= 0  SaturateOnIntegerOverflow=off  InputSameDT=off
  Signal_out : Outport
  wires:
  Mod2/1 -> Mux/4  "Theta_e"
  Derivative/1 -> Divide1/2
  Signal_In/1 -> Bus Selector/1
  Pole_Pairs2/1 -> Mod2/1
  Divide2/1 -> Sum2/2  "Te"
  Mod/1 -> Mux/3, Pole_Pairs2/1  "Theta_m"
  Sum2/1 -> Sum3/2
  Gain/1 -> Gain1/1, Derivative/1, Integrator/1, Pole_Pairs/1, Mux/1, Relational Operator/1, Switch/3  "Wm"
  Inertia/1 -> Divide1/1
  Mux/1 -> Signal_out/1  "Signal_out"
  Gain1/1 -> Sum2/1  "Bwm"
  Pole_Pairs/1 -> Mux/2  "We"
  Integrator/1 -> Mod/1
  PI2/1 -> Mod/2
  PI1/1 -> Mod2/2
  Bus Selector/2 -> Product/1  "<dSimEs>"
  Divide1/1 -> Sum3/1
  Sum3/1 -> Mux/5  "TL"
  Sum1/1 -> Divide2/1  "Pe"
  Product/1 -> Sum1/1
  Bus Selector/3 -> Product/2  "<dSimIabc>"
  Bus Selector/1 -> Gain/1  "<S_Load>"
  Constant/1 -> Relational Operator/2
  Relational Operator/1 -> Switch/2
  Constant1/1 -> Switch/1
  Switch/1 -> Divide2/2

== system a01_SimTurret/Turret/SimFtnServoMotor/DynamoSystem/TorqueMode ==
  note: TL
  note: B
  note: J
  Signal_In : Inport
  Bus Selector : BusSelector  OutputSignals=S_Load,T_Load,dSimEs,dSimIabc
  Constant : Constant  Value=0  OutDataTypeStr=double
  Constant1 : Constant  Value=eps  OutDataTypeStr=double
  Divide : Product  Inputs=*/
  Divide1 : Product  Inputs=*/
  Gain2 : Gain  Gain=MtrPar.B
  Integrator : Integrator  InitialCondition=Sim.Init.Wm / 30 *pi + eps
  Integrator2 : Integrator  InitialCondition=Sim.Init.Elec_Angle / 180 * pi / MtrPar.Poles * 2
  Mech2 : Constant  Value=MtrPar.J
  Mod : Math  Operator=mod  SignedPower=on
  Mod2 : Math  Operator=mod  SignedPower=on
  Mux : Mux  Inputs=5
  PI1 : Constant  Value=2*pi
  PI2 : Constant  Value=2*pi
  Pole_Pairs : Gain  Gain=MtrPar.PolePairs
  Pole_Pairs2 : Gain  Gain=MtrPar.PolePairs
  Product2 : Product
  Relational Operator : RelationalOperator  Operator===  OutDataTypeStr=boolean  RndMeth=Simplest  InputSameDT=off
  Sum : Sum  Inputs=--+
  Sum1 : Sum  Inputs=+
  Switch : Switch  Criteria=u2 ~= 0  SaturateOnIntegerOverflow=off  InputSameDT=off
  Terminator : Terminator
  Signal_out : Outport
  wires:
  Sum/1 -> Divide/1  "Teff"
  Mod/1 -> Mux/3, Pole_Pairs2/1  "Theta_m"
  Divide1/1 -> Sum/3, Mux/5  "Te"
  Integrator/1 -> Integrator2/1, [Wm], Mux/1, Gain2/1, Pole_Pairs/1  "Wm"
  Integrator2/1 -> Mod/1
  Gain2/1 -> Sum/1  "BWm"
  PI2/1 -> Mod/2
  Pole_Pairs2/1 -> Mod2/1  "Pst"
  Mod2/1 -> Mux/4  "Theta_e"
  Pole_Pairs/1 -> Mux/2  "We"
  PI1/1 -> Mod2/2
  Divide/1 -> Integrator/1  "dW/dt"
  Bus Selector/2 -> Sum/2  "<T_Load>"
  Signal_In/1 -> Bus Selector/1
  Mux/1 -> Signal_out/1  "Signal_out"
  Bus Selector/1 -> Terminator/1  "<S_Load>"
  Mech2/1 -> Divide/2
  Constant1/1 -> Switch/1
  Switch/1 -> Divide1/2  "Wm"
  Product2/1 -> Sum1/1  "Pe"
  Relational Operator/1 -> Switch/2
  Sum1/1 -> Divide1/1  "PeSum"
  [Wm] -> Switch/3, Relational Operator/1
  Constant/1 -> Relational Operator/2
  Bus Selector/3 -> Product2/1  "<dSimEs>"
  Bus Selector/4 -> Product2/2  "<dSimIabc>"

== system a01_SimTurret/Turret/SimFtnServoMotor/Nftn_EncOut/mod ==
  sThetaIntegIn : Inport
  Add1 : Sum
  Constant1 : Constant  Value=0  OutDataTypeStr=single
  Constant2 : Constant  Value=2*pi
  Relational Operator2 : RelationalOperator  Operator=>  OutDataTypeStr=boolean  InputSameDT=off
  RelationalOperator1 : RelationalOperator  Operator=>  OutDataTypeStr=boolean  InputSameDT=off
  Sum1 : Sum  Inputs=+-
  Switch2 : Switch  Criteria=u2 ~= 0  SaturateOnIntegerOverflow=off  InputSameDT=off
  Switch3 : Switch  Criteria=u2 ~= 0  SaturateOnIntegerOverflow=off  InputSameDT=off
  sThetaIntegOut : Outport  VectorParamsAs1DForOutWhenUnconnected=off
  wires:
  sThetaIntegIn/1 -> Switch2/1, RelationalOperator1/1, Add1/1
  Constant1/1 -> RelationalOperator1/2
  RelationalOperator1/1 -> Switch2/2
  Add1/1 -> Switch2/3
  Constant2/1 -> Add1/2, Relational Operator2/2, Sum1/2
  Switch2/1 -> Switch3/3, Relational Operator2/1, Sum1/1
  Relational Operator2/1 -> Switch3/2
  Sum1/1 -> Switch3/1
  Switch3/1 -> sThetaIntegOut/1

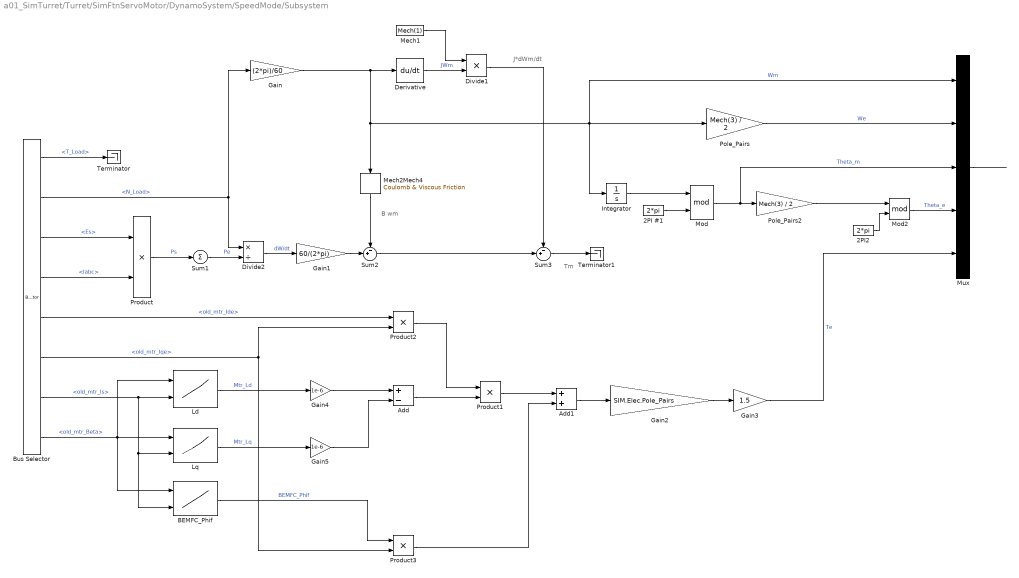
== system a01_SimTurret/Turret/SimFtnServoMotor/DynamoSystem/SpeedMode/Subsystem ==
  note: Tm
  note: J*dWm/dt
  note: B wm
  2PI #1 : Constant  Value=2*pi
  2PI2 : Constant  Value=2*pi
  Add : Sum  Inputs=+-
  Add1 : Sum
  BEMFC_Phif : Lookup_n-D  BreakpointsForDimension1=SIM.Arry.Ke_BrkP1_Beta  BreakpointsForDimension2=SIM.Arry.Ke_BrkP2_Is  Table=SIM.Arry.Ke_TableData_BEMFC_Phif  RemoveProtectionInput=on  InternalRulePriority=Speed  RndMeth=Simplest
      settings: InputPortMap=u0,u1
  Bus Selector : BusSelector  OutputSignals=T_Load,N_Load,Es,Iabc,signal5.old_mtr_Ide,signal5.old_mtr_Iqe,signal5.old_mtr_Is,signal5.old_mtr_Beta
  Derivative : Derivative
  Divide1 : Product  Inputs=**
  Divide2 : Product  Inputs=*/
  Gain : Gain  Gain=(2*pi)/60
  Gain1 : Gain  Gain=60/(2*pi)
  Gain2 : Gain  Gain=SIM.Elec.Pole_Pairs
  Gain3 : Gain  Gain=1.5
  Gain4 : Gain  Gain=1e-6
  Gain5 : Gain  Gain=1e-6
  Integrator : Integrator
  Ld : Lookup_n-D  BreakpointsForDimension1=SIM.Arry.Ke_BrkP1_Beta  BreakpointsForDimension2=SIM.Arry.Ke_BrkP2_Is  Table=SIM.Arry.Ke_TableData_Ld  RemoveProtectionInput=on  InternalRulePriority=Speed  RndMeth=Simplest
      settings: InputPortMap=u0,u1
  Lq : Lookup_n-D  BreakpointsForDimension1=SIM.Arry.Ke_BrkP1_Beta  BreakpointsForDimension2=SIM.Arry.Ke_BrkP2_Is  Table=SIM.Arry.Ke_TableData_Lq  RemoveProtectionInput=on  InternalRulePriority=Speed  RndMeth=Simplest
      settings: InputPortMap=u0,u1
  Mech1 : Constant  Value=Mech(1)
  Mech2Mech4 : simulink/Discontinuities/Coulomb & Viscous Friction  offset=Mech(4)  gain=Mech(2)
  Mod : Math  Operator=mod  SignedPower=on
  Mod2 : Math  Operator=mod  SignedPower=on
  Mux : Mux  Inputs=5
  Pole_Pairs : Gain  Gain=Mech(3) / 2
  Pole_Pairs2 : Gain  Gain=Mech(3) / 2
  Product{,1..3} (4 alike) : Product
  Sum1 : Sum  Inputs=+
  Sum2 : Sum  Inputs=-+|
  Sum3 : Sum  Inputs=-+|
  Terminator : Terminator
  Terminator1 : Terminator
  wires:
  Gain3/1 -> Mux/5  "Te"
  Bus Selector/5 -> Product2/1  "<old_mtr_Ide>"
  Mech1/1 -> Divide1/1
  Add1/1 -> Gain2/1
  BEMFC_Phif/1 -> Product3/1  "BEMFC_Phif"
  Add/1 -> Product1/2
  Divide2/1 -> Gain1/1  "dW/dt"
  Lq/1 -> Gain5/1  "Mtr_Lq"
  Product3/1 -> Add1/2
  Product1/1 -> Add1/1
  Sum2/1 -> Sum3/2
  Bus Selector/1 -> Terminator/1  "<T_Load>"
  Gain4/1 -> Add/1
  Gain2/1 -> Gain3/1
  Divide1/1 -> Sum3/1
  2PI2/1 -> Mod2/2
  Gain5/1 -> Add/2
  Product2/1 -> Product1/1
  Ld/1 -> Gain4/1  "Mtr_Ld"
  Bus Selector/7 -> BEMFC_Phif/2, Lq/2, Ld/2  "<old_mtr_Is>"
  Pole_Pairs/1 -> Mux/2  "We"
  Sum3/1 -> Terminator1/1
  Product/1 -> Sum1/1  "Ps"
  Integrator/1 -> Mod/1
  Mux/1 -> ?
  Bus Selector/8 -> BEMFC_Phif/1, Lq/1, Ld/1  "<old_mtr_Beta>"
  Derivative/1 -> Divide1/2  "JWm"
  2PI #1/1 -> Mod/2
  Sum1/1 -> Divide2/2  "Pe"
  Bus Selector/4 -> Product/2  "<Iabc>"
  Mech2Mech4/1 -> Sum2/1
  Bus Selector/3 -> Product/1  "<Es>"
  Gain/1 -> Mech2Mech4/1, Integrator/1, Pole_Pairs/1, Mux/1, Derivative/1  "Wm"
  Bus Selector/2 -> Gain/1, Divide2/1  "<N_Load>"
  ? -> Bus Selector/1
  Mod/1 -> Pole_Pairs2/1, Mux/3  "Theta_m"
  Bus Selector/6 -> Product2/2, Product3/2  "<old_mtr_Iqe>"
  Gain1/1 -> Sum2/2
  Mod2/1 -> Mux/4  "Theta_e"
  Pole_Pairs2/1 -> Mod2/1

== stateflow chart a01_SimTurret/BSW_CAN/Chart_CanTxTimer1 ==
  (default) -> (junction 2)
  (junction 2) -> (junction 3) [order 1] : [i32CntArrNo >= i32MaxCntArrNo]
  (junction 2) -> (junction 13) [order 2] : {
      | i32CntArrNo = i32CntArrNo + Const_i32Step;
      | }
  (junction 3) -> (junction 4) : {
      | i32CntArrNo = Const_i32InitCnt;
      | }
  (junction 4) -> (junction 13)
  (junction 13) -> (junction 16)
  data: i32CntArrNo output int32 =9; Const_i32InitCnt constant int32 =0; i32MaxCntArrNo input int32; Const_i32Step constant int32 =1

== stateflow chart a01_SimTurret/BSW_GVAL/Chart_CalSingleTurnDeParts ==
  (default) -> (junction 1)
  (junction 1) -> (junction 3) : {
      | mEnc_uABS0 = uint16(mSimPst_u32EncCnt & 0x000000FF);
      | mEnc_uABS1 = uint16((mSimPst_u32EncCnt>>8) & 0x000000FF);
      | mEnc_uABS2 = uint16((mSimPst_u32EncCnt>>16) & 0x000000FF);
      | }
  (junction 3) -> (junction 11) : {
      | mEnc_uABM0 = uint16(mSimPst_u16EncMultiCnt & 0x00FF);
      | mEnc_uABM1 = uint16((mSimPst_u16EncMultiCnt>>8) & 0x00FF);
      | mEnc_uABM2 = Cnst_u16Zero;
      | }
  data: mEnc_uABS0 output uint16; mEnc_uABS1 output uint16; mEnc_uABS2 output uint16; mSimPst_u32EncCnt input; mSimPst_u16EncMultiCnt input; Cnst_u16Zero constant uint16 =0; mEnc_uABM0 output uint16; mEnc_uABM1 output uint16; mEnc_uABM2 output uint16

== stateflow chart a01_SimTurret/Turret/SimFtnServoMotor/Nftn_EncOut/Chart_EncOut ==
  (default) -> (junction 9) : {
      | tmp = i32EncSingleCntZ - i32EncSingleCnt;
      | }
  (junction 9) -> (junction 10) [order 1] : [tmp > Cnst_i32HalfSingleCnt]
  (junction 10) -> (junction 12) : {
      | i32EncMultiCnt = i32EncMultiCnt + 1;
      | }
  (junction 9) -> (junction 16) [order 2]
  (junction 16) -> (junction 18) [order 1] : [tmp < -Cnst_i32HalfSingleCnt]
  (junction 16) -> (junction 11) [order 2] : % No Action
  (junction 18) -> (junction 19) : {
      | i32EncMultiCnt = i32EncMultiCnt - 1;
      | }
  (junction 12) -> (junction 19)
  (junction 19) -> (junction 11)
  (junction 11) -> (junction 29)
  (junction 29) -> (junction 30) [order 1] : [i32EncMultiCnt > Cnst_i32HalfSingleCnt]
  (junction 30) -> (junction 32) : {
      | i32EncMultiCnt = i32EncMultiCnt - Cnst_i32HalfSingleCnt - 1;
      | }
  (junction 29) -> (junction 34) [order 2]
  (junction 34) -> (junction 42) [order 1] : [i32EncMultiCnt < Cnst_i32Zero]
  (junction 34) -> (junction 38) [order 2] : % No Action
  (junction 42) -> (junction 41) : {
      | i32EncMultiCnt = i32EncMultiCnt + Cnst_i32HalfSingleCnt + 1;
      | }
  (junction 32) -> (junction 41)
  (junction 41) -> (junction 38)
  (junction 38) -> (junction 62) : {
      | i32EncSingleCntZ = i32EncSingleCnt;
      | }
  data: i32EncSingleCnt input; i32EncMultiCnt output int32 =65530; Cnst_i32HalfSingleCnt constant int32 =65535; Cnst_i32Zero constant int32 =0; tmp local int32; i32EncSingleCntZ output
